simulink model "linsys1_mdl"  (R2022b)
settings: Solver=ode4  StartTime=0.0  StopTime=3  FixedStep=.01  MaxStep=.01  RelTol=1e-3
values from neighbouring files (symbols this model uses):
  A = exp(-a*Ts)    [RunMeFirst.m]    (also in linsys1.m = -a)
  B = 1    [RunMeFirst.m]    (also in linsys1.m = b)
  C = 1    [RunMeFirst.m]    (also in linsys1.m)
  R = .2    (= 0.2)    [RunMeFirst.m]    (also in linsys1.m = 0.5)
  Ts = .05    (= 0.05)    [RunMeFirst.m]    (also in linsys1.m = 0.1)
undefined symbols (not defined in the file or in its folder): DiscIntNeverNeededParam
libraries: simulink x3
settings Model: Creator=hp_desktop  LastModifiedBy=hp_desktop

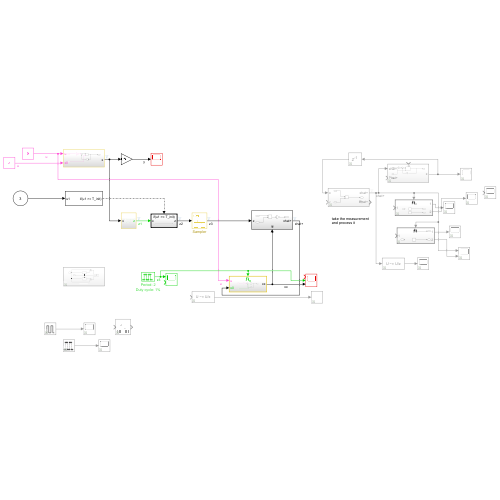
[thumbnail: Simulink's stored preview of the top-level diagram]
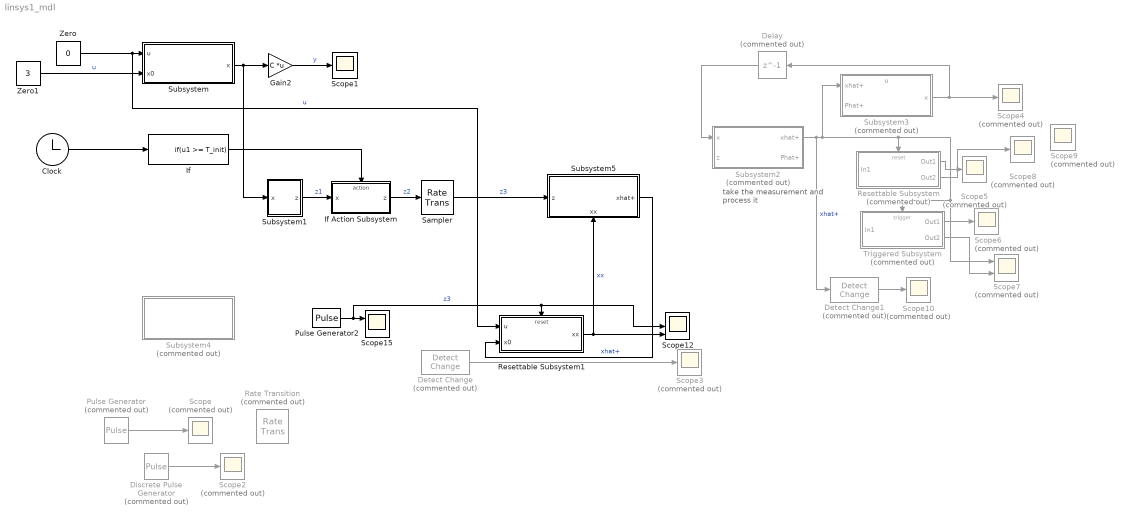
== system linsys1_mdl ==
  note: take the measurement
      | and process it
  Clock : Clock
  Delay : Delay  Commented=on  DelayLength=1
  Detect Change : simulink/Logic and Bit Operations/Detect Change  Commented=on  vinit=0  OutDataTypeStr=boolean
  Detect Change1 : simulink/Logic and Bit Operations/Detect Change  Commented=on  vinit=0  OutDataTypeStr=uint8
  Discrete Pulse Generator : DiscretePulseGenerator  Commented=on
  Gain2 : Gain  Gain=C  Multiplication=Matrix(K*u)
  If : If  IfExpression=u1 >= T_init  ShowElse=off
  If Action Subsystem : Subsystem  TreatAsAtomicUnit=on
  Pulse Generator : DiscretePulseGenerator  Commented=on  PulseType=Time based  Period=1  PulseWidth=5
  Pulse Generator2 : DiscretePulseGenerator  SampleTime=.1
      settings: AttributesFormatString=Period: %<period>\nDuty cycle: %<pulsewidth>%
  Rate Transition : RateTransition  Commented=on
  Resettable Subsystem : Subsystem  Commented=on  TreatAsAtomicUnit=on
  Resettable Subsystem1 : Subsystem  TreatAsAtomicUnit=on
  Sampler : RateTransition  OutPortSampleTime=Ts
  Scope{,2..6,8..10} (9 alike) : Scope  Commented=on
  Scope1 : Scope
  Scope12 : Scope  NumInputPorts=3
  Scope15 : Scope  NumInputPorts=2
  Scope7 : Scope  Commented=on  NumInputPorts=2
  Subsystem : Subsystem
  Subsystem1 : Subsystem
  Subsystem2 : Subsystem  Commented=on
  Subsystem3 : Subsystem  Commented=on
      settings: PortSchema="{\"entries\":[{\"content\":{\"sides\":[{\"content\":{\"connectorIds\":[\"In1\",\"In2\"]},\"type\":\"ConnectorPlacement.EquallySpacedRectSide\",\"uuid\":\"098bb33a-295b-4037-94a1-aad71dea8bca\"},{\"content\":{\"connectorIds\":[\"Out1\"],\"side\":\"RIGHT\"},\"type\":\"ConnectorPlacement.EquallySpacedRectSide\",\"uuid\":\"dacc0f14-46b8-43e5-9194-363d38e9a812\"},{\"content\":{\"connectorIds\":[\"In3\"],\"side\":\"TOP\"},\"type\":\"ConnectorPlacement.EquallySpacedRectSide\",\"uuid\":\"2d6ed1d8-1ca0-472f-a83e-22717d75ce74\"}]},\"type\":\"ConnectorPlacement.EquallySpacedConnector\",\"uuid\":\"9911ff5e-034c-4b18-8486-9a9946e68fe4\"}],\"packageUris\":[\"http://schema.mathworks.com/mf0/Connector/R2020b\"],\"version\":\"1.0\"}"
  Subsystem4 : Subsystem  Commented=on
  Subsystem5 : Subsystem
      settings: PortSchema="{\"entries\":[{\"content\":{\"sides\":[{\"content\":{\"connectorIds\":[\"In1\"]},\"type\":\"ConnectorPlacement.EquallySpacedRectSide\",\"uuid\":\"cdc9ee4c-2332-4df4-a9ed-8b1a0f764cb5\"},{\"content\":{\"connectorIds\":[\"Out1\"],\"side\":\"RIGHT\"},\"type\":\"ConnectorPlacement.EquallySpacedRectSide\",\"uuid\":\"425f78b2-1c90-4e1b-86c0-f70016492d4b\"},{\"content\":{\"connectorIds\":[],\"side\":\"TOP\"},\"type\":\"ConnectorPlacement.EquallySpacedRectSide\",\"uuid\":\"996d94b4-9ccf-4a7a-bdc0-fe5c726dc8d7\"},{\"content\":{\"connectorIds\":[\"In2\"],\"side\":\"BOTTOM\"},\"type\":\"ConnectorPlacement.EquallySpacedRectSide\",\"uuid\":\"5b3e15c4-1826-410c-96e5-ab3e919096d2\"}]},\"type\":\"ConnectorPlacement.EquallySpacedConnector\",\"uuid\":\"982a7e94-c813-4d4f-ba49-60caf9c845b1\"}],\"packageUris\":[\"http://schema.mathworks.com/mf0/Connector/R2020b\"],\"version\":\"1.0\"}"
  Triggered Subsystem : Subsystem  Commented=on  TreatAsAtomicUnit=on
  Zero : Constant  Value=0  OutDataTypeStr=Inherit: Inherit via back propagation
  Zero1 : Constant  Value=3  OutDataTypeStr=Inherit: Inherit via back propagation
  wires:
  Gain2/1 -> Scope1/1  "y"
  Pulse Generator/1 -> Scope/1
  Zero/1 -> Resettable Subsystem1/1(u), Subsystem/1(u)  "u"
  Subsystem/1(x) -> Subsystem1/1(x), Gain2/1
  Discrete Pulse Generator/1 -> Scope2/1
  Clock/1 -> If/1
  If/1 -> If Action Subsystem/Action
  Subsystem1/1(z) -> If Action Subsystem/1(x)  "z1"
  Zero1/1 -> Subsystem/2(x0)  "u"
  If Action Subsystem/1(z) -> Sampler/1  "z2"
  Detect Change/1 -> Scope3/1
  Subsystem2/1(xhat+) -> Scope7/1, Triggered Subsystem/Trigger, Resettable Subsystem/Reset, Subsystem3/1(xhat+), Detect Change1/1  "xhat+"
  Subsystem3/1(x) -> Scope4/1, Delay/1
  Delay/1 -> Subsystem2/1(x)
  Resettable Subsystem/1(Out1) -> Scope5/1
  Triggered Subsystem/1(Out1) -> Scope6/1
  Triggered Subsystem/2(Out2) -> Scope7/2
  Resettable Subsystem/2(Out2) -> Scope8/1
  Detect Change1/1 -> Scope10/1
  Resettable Subsystem1/1(xx) -> Scope12/3, Subsystem5/2(xx)  "xx"
  Pulse Generator2/1 -> Scope12/2, Resettable Subsystem1/Reset, Scope15/1  "z3"
  Sampler/1 -> Subsystem5/1(z)  "z3"
  Subsystem5/1(xhat+) -> Resettable Subsystem1/2(x0)  "xhat+"

== system linsys1_mdl/If Action Subsystem ==
  x : Inport
  Action Port : ActionPort  ActionPortLabel=if(u1 >= T_init)
  z : Outport  OutputWhenDisabled=reset  InitialOutput=0
  wires:
  x/1 -> z/1

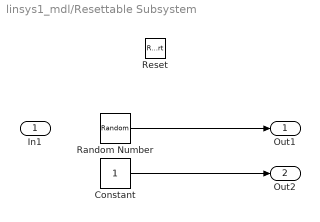
== system linsys1_mdl/Resettable Subsystem ==
  In1 : Inport
  Reset : ResetPort  DisableCoverage=on  ResetTriggerType=either
  Constant : Constant
  Random Number : RandomNumber  SampleTime=0.1
  Out1 : Outport
  Out2 : Outport  Port=2
  wires:
  Random Number/1 -> Out1/1
  Constant/1 -> Out2/1

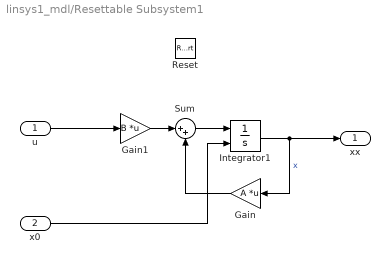
== system linsys1_mdl/Resettable Subsystem1 ==
  u : Inport
  x0 : Inport  Port=2
  Reset : ResetPort  DisableCoverage=on  ResetTriggerType=either
  Gain : Gain  Gain=A  Multiplication=Matrix(K*u)
  Gain1 : Gain  Gain=B  Multiplication=Matrix(K*u)
  Integrator1 : Integrator  InitialConditionSource=external
  Sum : Sum  Inputs=|++
  xx : Outport
  wires:
  u/1 -> Gain1/1
  Integrator1/1 -> xx/1, Gain/1  "x"
  x0/1 -> Integrator1/2
  Sum/1 -> Integrator1/1
  Gain/1 -> Sum/2
  Gain1/1 -> Sum/1

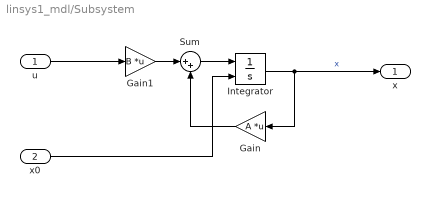
== system linsys1_mdl/Subsystem ==
  u : Inport
  x0 : Inport  Port=2
  Gain : Gain  Gain=A  Multiplication=Matrix(K*u)
  Gain1 : Gain  Gain=B  Multiplication=Matrix(K*u)
  Integrator : Integrator  InitialConditionSource=external
  Sum : Sum  Inputs=|++
  x : Outport
  wires:
  Integrator/1 -> x/1, Gain/1  "x"
  Sum/1 -> Integrator/1
  u/1 -> Gain1/1
  Gain/1 -> Sum/2
  Gain1/1 -> Sum/1
  x0/1 -> Integrator/2

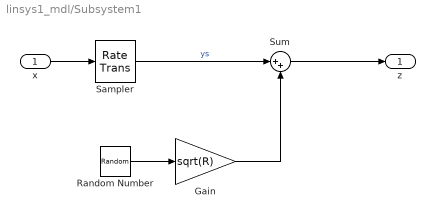
== system linsys1_mdl/Subsystem1 ==
  x : Inport
  Gain : Gain  Gain=sqrt(R)
  Random Number : RandomNumber  SampleTime=Ts  VectorParams1D=off
  Sampler : RateTransition  OutPortSampleTime=Ts
  Sum : Sum  Inputs=|++
  z : Outport
  wires:
  Random Number/1 -> Gain/1
  x/1 -> Sampler/1
  Sampler/1 -> Sum/1  "ys"
  Gain/1 -> Sum/2
  Sum/1 -> z/1

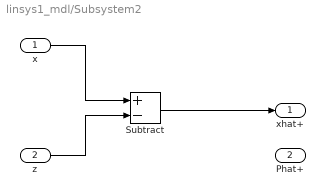
== system linsys1_mdl/Subsystem2 ==
  x : Inport
  z : Inport  Port=2
  Subtract : Sum  Inputs=+-
  xhat+ : Outport
  Phat+ : Outport  Port=2
  wires:
  x/1 -> Subtract/1
  z/1 -> Subtract/2
  Subtract/1 -> xhat+/1

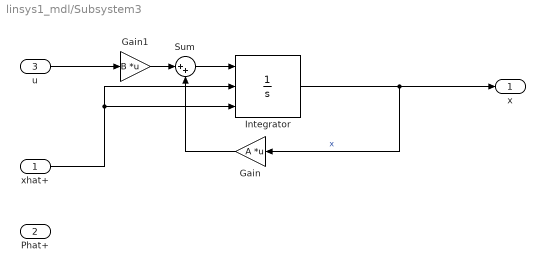
== system linsys1_mdl/Subsystem3 ==
  xhat+ : Inport
  Phat+ : Inport  Port=2
  u : Inport  Port=3
  Gain : Gain  Gain=A  Multiplication=Matrix(K*u)
  Gain1 : Gain  Gain=B  Multiplication=Matrix(K*u)
  Integrator : Integrator  ExternalReset=either  InitialConditionSource=external
  Sum : Sum  Inputs=|++
  x : Outport
  wires:
  Gain1/1 -> Sum/1
  Sum/1 -> Integrator/1
  xhat+/1 -> Integrator/2, Integrator/3
  Gain/1 -> Sum/2
  Integrator/1 -> x/1, Gain/1  "x"
  u/1 -> Gain1/1

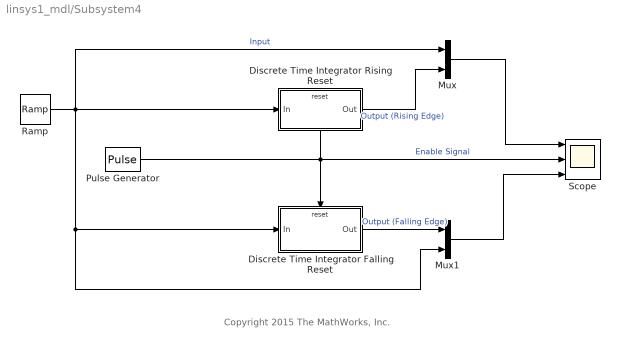
== system linsys1_mdl/Subsystem4 ==
  note: Copyright 2015 The MathWorks, Inc.
  Discrete Time Integrator Falling Reset : Subsystem  TreatAsAtomicUnit=on
  Discrete Time Integrator Rising Reset : Subsystem  TreatAsAtomicUnit=on
  Mux : Mux  Inputs=2
  Mux1 : Mux  Inputs=2
  Pulse Generator : DiscretePulseGenerator  Period=40  PulseWidth=20  SampleTime=.1
      settings: AttributesFormatString=Period: %<period>\nDuty cycle: %<pulsewidth>%
  Ramp : simulink/Sources/Ramp  slope=0.5  start=0  InitialOutput=1
  Scope : Scope  NumInputPorts=3
      settings: StartFcn=open_system(gcbh)
  wires:
  Ramp/1 -> Mux/1, Discrete Time Integrator Rising Reset/1(In), Mux1/2, Discrete Time Integrator Falling Reset/1(In)  "Input"
  Discrete Time Integrator Falling Reset/1(Out) -> Mux1/1  "Output (Falling Edge)"
  Mux/1 -> Scope/1
  Discrete Time Integrator Rising Reset/1(Out) -> Mux/2  "Output (Rising Edge)"
  Mux1/1 -> Scope/3
  Pulse Generator/1 -> Scope/2, Discrete Time Integrator Falling Reset/Reset, Discrete Time Integrator Rising Reset/Reset  "Enable Signal"

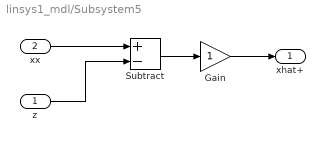
== system linsys1_mdl/Subsystem5 ==
  z : Inport
  xx : Inport  Port=2
  Gain : Gain
  Subtract : Sum  Inputs=+-
  xhat+ : Outport
  wires:
  Subtract/1 -> Gain/1
  z/1 -> Subtract/2
  xx/1 -> Subtract/1
  Gain/1 -> xhat+/1

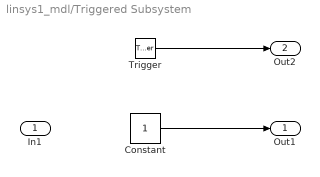
== system linsys1_mdl/Triggered Subsystem ==
  In1 : Inport
  Trigger : TriggerPort  TriggerType=either  VariantControl=(inherit)  ShowOutputPort=on  InitialTriggerSignalState=zero
  Constant : Constant
  Out1 : Outport  InitialOutput=0
  Out2 : Outport  Port=2  InitialOutput=0
  wires:
  Trigger/1 -> Out2/1
  Constant/1 -> Out1/1

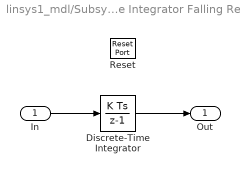
== system linsys1_mdl/Subsystem4/Discrete Time Integrator Falling Reset ==
  In : Inport  SampleTime=.1
  Reset : ResetPort  DisableCoverage=on  ResetTriggerType=falling
  Discrete-Time Integrator : DiscreteIntegrator  SampleTime=.1  ICPrevOutput=DiscIntNeverNeededParam  ICPrevScaledInput=DiscIntNeverNeededParam
  Out : Outport  VectorParamsAs1DForOutWhenUnconnected=off
  wires:
  Discrete-Time Integrator/1 -> Out/1
  In/1 -> Discrete-Time Integrator/1

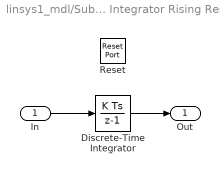
== system linsys1_mdl/Subsystem4/Discrete Time Integrator Rising Reset ==
  In : Inport  SampleTime=0.1
  Reset : ResetPort  DisableCoverage=on
  Discrete-Time Integrator : DiscreteIntegrator  SampleTime=-1  ICPrevOutput=DiscIntNeverNeededParam  ICPrevScaledInput=DiscIntNeverNeededParam
  Out : Outport  OutputWhenDisabled=reset  InitialOutput=0  VectorParamsAs1DForOutWhenUnconnected=off
  wires:
  In/1 -> Discrete-Time Integrator/1
  Discrete-Time Integrator/1 -> Out/1
